simulink model "HVAC_Model"  (R2017b)
settings: Solver=VariableStepAuto  StartTime=0.0  StopTime=260  RelTol=1e-3
model workspace (MAT data in the model file):
  H_Speed = 3600
  H_limit = 2500
  L_limit = 0
  inputVoltage = 5
  nBitConverter = 10
undefined symbols (not defined in the file): sigbuilder_block
libraries: simulink x1
settings Model: Creator=ECoDe_user11  LastModifiedBy=ECoDe_user11
settings DebuggingCC: SignalInfNanChecking=warning  ParameterUnderflowMsg=warning  UniqueDataStoreMsg=warning
settings ConfigComp: CovEnable=on  RecordCoverage=on  CovMetricSettings=dcmwe  CovModelRefEnable=on

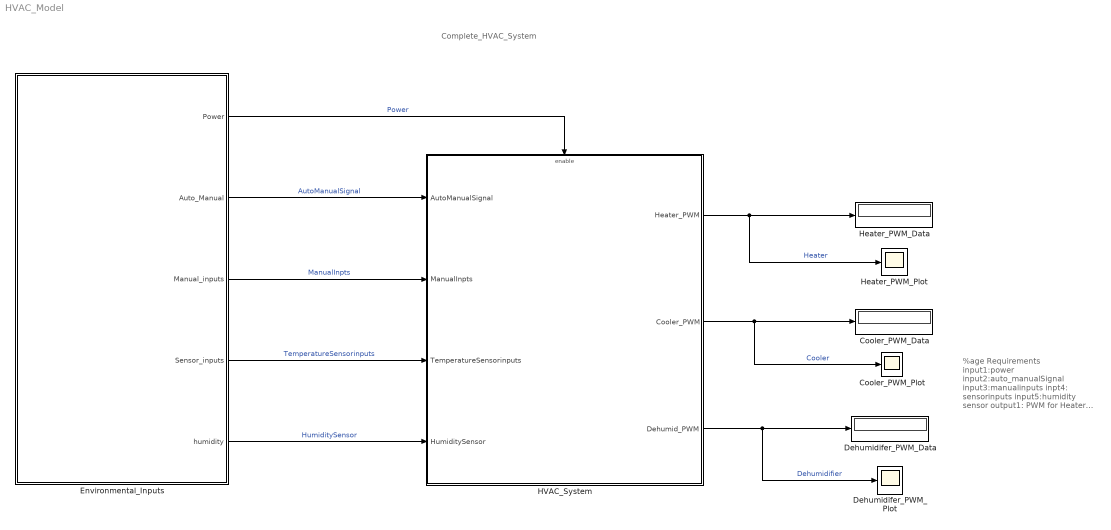
== system HVAC_Model ==
  note: Complete_HVAC_System
  note: %age Requirements
      |
      | input1:power
      | input2:auto_manualSignal
      | input3:manualinputs
      | inpt4: sensorinputs
      | input5:humidity sensor
      | output1: PWM for Heater
      | output1: PWM for Cooler
      | output1: PWM for Dehumidifier
  Cooler_PWM_Data : Display
  Cooler_PWM_Plot : Scope
  Dehumidifer_PWM_Data : Display
  Dehumidifer_PWM_Plot : Scope
  Environmental_Inputs : Subsystem  Tag=STV Subsys  LoadFcn=sigbuilder_block('load',[437.25 159 550.5 363.75 ]);  StartFcn=sigbuilder_block('start');  StopFcn=sigbuilder_block('stop');  ClipboardFcn=sigbuilder_block('clipboard');  mask(Sigbuilder block){tuvar=[0:10]}
      mask help: Simulink:masks:SigbuilderBlock_MD
      mask init:
      | if ~strcmp(get_param(bdroot(gcbh),'SimulationStatus'),'stopped') tuvar = sigbuilder_block('maskInit'); end
      settings: CopyFcn=sigbuilder_block('copy');  DeleteFcn=sigbuilder_block('delete');  ModelCloseFcn=sigbuilder_block('modelClose');  PreSaveFcn=sigbuilder_block('preSave');  PauseFcn=sigbuilder_block('pause');  ContinueFcn=sigbuilder_block('continue');  NameChangeFcn=sigbuilder_block('namechange');  OpenFcn=sigbuilder_block('open',[437.25 159 550.5 363.75 ]);  CloseFcn=sigbuilder_block('close');
      mask Display: plot(0, 0, 100, 100,[2, 2, 32, 32, 2], [68, 8, 8, 68, 68],[32, 2], [38, 38], [32, 19, 2],[53, 60, 44], [32, 17, 17, 2],[16, 16, 31, 31]);txt = getActiveGroup(gcbh);text(2, 100, txt,'verticalAlignment', 'top');
  HVAC_System : Subsystem
  Heater_PWM_Data : Display
  Heater_PWM_Plot : Scope
  wires:
  Environmental_Inputs/2(Auto_Manual) -> HVAC_System/1(AutoManualSignal)  "AutoManualSignal"
  Environmental_Inputs/3(Manual_inputs) -> HVAC_System/2(ManualInpts)  "ManualInpts"
  Environmental_Inputs/4(Sensor_inputs) -> HVAC_System/3(TemperatureSensorinputs)  "TemperatureSensorinputs"
  Environmental_Inputs/1(Power) -> HVAC_System/Enable  "Power"
  HVAC_System/1(Heater_PWM) -> Heater_PWM_Plot/1, Heater_PWM_Data/1  "Heater"
  HVAC_System/3(Dehumid_PWM) -> Dehumidifer_PWM_Plot/1, Dehumidifer_PWM_Data/1  "Dehumidifier"
  Environmental_Inputs/5(humidity) -> HVAC_System/4(HumiditySensor)  "HumiditySensor"
  HVAC_System/2(Cooler_PWM) -> Cooler_PWM_Plot/1, Cooler_PWM_Data/1  "Cooler"

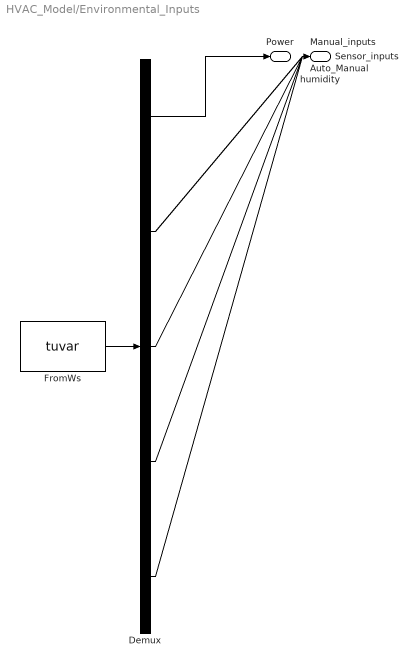
== system HVAC_Model/Environmental_Inputs ==
  Demux : Demux  Tag=STV Demux  Outputs=5
  FromWs : FromWorkspace  Tag=STV FromWs  VariableName=tuvar  SampleTime=0
      SigBuilderData=|
      | common.afterFinalStr = 'Extrapolate'
      | common.sampleTime = 0
      | dataSet.timeRange = [0 258]
      | dataSet.name = 'Sheet1'
      | sbobj.Name = 'Signal Builder'
      | sbobj.Groups.Name = 'Sheet1'
      | sbobj.Groups.Signals(1).Name = 'Power'
      | sbobj.Groups.Signals(1).XData = [0 1 2 3 4 5 6 7 8 9 10 11 12 13 14 15 16 17 18 19 20 21 22 23 24 25 26 27 28 29 30 31 32 33 34 35 36 37 38 39 40 41 42 43 44 45 46 47 48 49 50 51 52 53 54 55 56 57 58 59 60 61 62 63 64 65 66 67 68 69 70 71 72 73 74 75 76 77 78 79 80 81 82 83 84 85 86 87 88 89 90 91 92 93 94 95 96 97 98 99 100 101 102 103 104 105 106 107 108 109 110 111 112 113 114 115 116 117 118 119 120 121 122 123 124 125 126 127 128 129 130 131 132 133 134 135 136 137 138 139 140 141 142 143 144 145 146 147 148 149 150 151 152 153 154 155 156 157 158 159 160 161 162 163 164 165 166 167 168 169 170 171 172 173 174 175 176 177 178 179 180 181 182 183 184 185 186 187 188 189 190 191 192 193 194 195 196 197 198 199 200 201 202 203 204 205 206 207 208 209 210 211 212 213 214 215 216 217 218 219 220 221 222 223 224 225 226 227 228 229 230 231 232 233 234 235 236 237 238 239 240 241 242 243 244 245 246 247 248 249 250 251 252 253 254 255 256 257 258]
      | sbobj.Groups.Signals(1).YData = [1 1 1 1 1 1 1 1 1 1 1 1 1 1 1 1 1 1 1 1 1 1 1 1 1 1 1 1 1 1 1 1 1 1 1 1 1 1 1 1 1 1 1 1 1 1 1 1 1 1 1 1 1 1 1 1 1 1 1 1 1 1 1 1 1 1 1 1 1 1 1 1 0 0 0 0 0 0 0 1 1 1 1 1 1 1 1 1 1 1 1 1 1 1 1 1 1 1 1 1 1 1 1 1 1 1 1 1 1 1 1 1 1 1 1 1 1 1 1 1 1 1 1 1 1 1 1 1 1 1 1 1 1 1 1 1 1 1 1 1 1 1 1 1 1 1 1 1 1 1 1 1 1 1 1 1 1 1 1 1 1 1 1 1 1 1 1 1 1 1 1 1 1 1 1 1 1 1 1 1 1 1 1 1 1 1 1 1 1 1 1 1 1 1 1 1 1 1 1 1 1 1 1 1 1 1 1 1 1 1 1 1 1 1 1 1 1 1 1 1 1 1 1 1 1 1 1 1 1 1 1 1 1 1 1 1 1 1 1 1 1 1 1 1 1 1 1 1 1 1 1 1 1 1 1 1 1 1 1]
      | sbobj.Groups.Signals(2).Name = 'Auto_Manual'
      | sbobj.Groups.Signals(2).XData = [0 1 2 3 4 5 6 7 8 9 10 11 12 13 14 15 16 17 18 19 20 21 22 23 24 25 26 27 28 29 30 31 32 33 34 35 36 37 38 39 40 41 42 43 44 45 46 47 48 49 50 51 52 53 54 55 56 57 58 59 60 61 62 63 64 65 66 67 68 69 70 71 72 73 74 75 76 77 78 79 80 81 82 83 84 85 86 87 88 89 90 91 92 93 94 95 96 97 98 99 100 101 102 103 104 105 106 107 108 109 110 111 112 113 114 115 116 117 118 119 120 121 122 123 124 125 126 127 128 129 130 131 132 133 134 135 136 137 138 139 140 141 142 143 144 145 146 147 148 149 150 151 152 153 154 155 156 157 158 159 160 161 162 163 164 165 166 167 168 169 170 171 172 173 174 175 176 177 178 179 180 181 182 183 184 185 186 187 188 189 190 191 192 193 194 195 196 197 198 199 200 201 202 203 204 205 206 207 208 209 210 211 212 213 214 215 216 217 218 219 220 221 222 223 224 225 226 227 228 229 230 231 232 233 234 235 236 237 238 239 240 241 242 243 244 245 246 247 248 249 250 251 252 253 254 255 256 257 258]
      | sbobj.Groups.Signals(2).YData = [0 0 0 0 0 0 0 0 0 0 0 0 0 0 0 0 0 0 0 0 0 1 1 1 1 1 1 1 1 1 1 1 1 1 1 1 1 1 1 1 1 1 1 1 1 1 1 1 1 1 1 1 1 1 1 1 1 1 1 1 1 1 1 1 1 1 1 1 1 1 1 1 1 1 1 0 0 0 0 1 1 1 1 1 1 1 1 1 1 1 1 1 1 1 1 1 1 1 1 1 1 1 1 1 1 1 1 1 1 1 1 1 1 1 1 1 1 1 1 1 1 1 1 1 1 1 1 1 1 1 1 1 1 1 1 1 1 1 1 1 1 1 1 1 1 1 1 1 1 1 1 1 1 1 1 1 1 1 1 1 1 1 1 1 1 1 1 1 1 1 1 1 1 1 1 1 1 1 1 1 1 1 1 1 1 1 1 1 1 1 1 1 1 1 1 1 1 1 1 1 1 1 1 1 1 1 1 1 1 1 1 1 1 1 1 1 1 1 1 1 1 1 1 1 1 1 1 1 1 1 1 1 1 1 1 1 1 1 1 1 1 1 1 1 1 1 1 1 1 1 1 1 1 1 1 1 1 1 1]
      | sbobj.Groups.Signals(3).Name = 'Manual_inputs'
      | sbobj.Groups.Signals(3).XData = [0 1 2 3 4 5 6 7 8 9 10 11 12 13 14 15 16 17 18 19 20 21 22 23 24 25 26 27 28 29 30 31 32 33 34 35 36 37 38 39 40 41 42 43 44 45 46 47 48 49 50 51 52 53 54 55 56 57 58 59 60 61 62 63 64 65 66 67 68 69 70 71 72 73 74 75 76 77 78 79 80 81 82 83 84 85 86 87 88 89 90 91 92 93 94 95 96 97 98 99 100 101 102 103 104 105 106 107 108 109 110 111 112 113 114 115 116 117 118 119 120 121 122 123 124 125 126 127 128 129 130 131 132 133 134 135 136 137 138 139 140 141 142 143 144 145 146 147 148 149 150 151 152 153 154 155 156 157 158 159 160 161 162 163 164 165 166 167 168 169 170 171 172 173 174 175 176 177 178 179 180 181 182 183 184 185 186 187 188 189 190 191 192 193 194 195 196 197 198 199 200 201 202 203 204 205 206 207 208 209 210 211 212 213 214 215 216 217 218 219 220 221 222 223 224 225 226 227 228 229 230 231 232 233 234 235 236 237 238 239 240 241 242 243 244 245 246 247 248 249 250 251 252 253 254 255 256 257 258]
      | sbobj.Groups.Signals(3).YData = [14 15 16 17 18 19 20 21 22 23 24 25 26 27 28 29 30 31 32 33 34 0 1 2 3 4 5 6 7 8 9 10 11 12 13 14 15 16 17 18 19 20 21 22 23 24 25 26 27 28 29 30 31 32 33 34 35 36 37 38 39 40 41 42 43 44 45 46 47 48 49 50 17 18 19 20 21 22 23 24 25 26 27 27 27 27 27 27 27 27 27 27 27 27 27 27 27 27 27 27 27 27 27 27 27 27 27 27 27 27 27 27 27 27 27 27 27 27 27 27 27 27 27 27 27 27 27 27 27 27 27 27 27 27 24 25 26 27 20 20 20 20 20 20 20 20 20 20 20 20 20 20 20 20 20 20 20 20 20 20 20 20 20 20 20 20 20 20 20 20 20 20 20 20 20 20 20 20 20 20 20 20 20 20 20 20 20 20 20 20 20 20 20 20 20 20 20 20 20 20 20 20 20 20 20 20 20 20 20 20 20 20 20 20 20 20 20 20 20 20 20 20 20 20 20 20 20 20 20 20 20 20 20 20 20 20 20 20 20 20 20 20 20 20 20 20 20 20 20 20 20 20 20 20 20 20 20 20 20]
      | sbobj.Groups.Signals(4).Name = 'Sensor_inputs'
      | sbobj.Groups.Signals(4).XData = [0 1 2 3 4 5 6 7 8 9 10 11 12 13 14 15 16 17 18 19 20 21 22 23 24 25 26 27 28 29 30 31 32 33 34 35 36 37 38 39 40 41 42 43 44 45 46 47 48 49 50 51 52 53 54 55 56 57 58 59 60 61 62 63 64 65 66 67 68 69 70 71 72 73 74 75 76 77 78 79 80 81 82 83 84 85 86 87 88 89 90 91 92 93 94 95 96 97 98 99 100 101 102 103 104 105 106 107 108 109 110 111 112 113 114 115 116 117 118 119 120 121 122 123 124 125 126 127 128 129 130 131 132 133 134 135 136 137 138 139 140 141 142 143 144 145 146 147 148 149 150 151 152 153 154 155 156 157 158 159 160 161 162 163 164 165 166 167 168 169 170 171 172 173 174 175 176 177 178 179 180 181 182 183 184 185 186 187 188 189 190 191 192 193 194 195 196 197 198 199 200 201 202 203 204 205 206 207 208 209 210 211 212 213 214 215 216 217 218 219 220 221 222 223 224 225 226 227 228 229 230 231 232 233 234 235 236 237 238 239 240 241 242 243 244 245 246 247 248 249 250 251 252 253 254 255 256 257 258]
      | sbobj.Groups.Signals(4).YData = [0.1 0.2 0.3 0.4 0.5 0.6 0.7 0.8 0.9 1 1.1 1.2 1.3 1.4 1.5 1.6 1.7 1.8 1.9 2 2.1 0.9 0.89 0.88 0.87 0.86 0.85 0.84 0.83 0.82 0.81 0.8 0.79 0.78 0.77 0.76 0.75 0.74 0.73 0.72 0.71 0.7 0.69 0.68 0.67 0.66 0.65 0.64 0.63 0.62 0.61 0.6 0.59 0.58 0.57 0.56 0.55 0.54 0.53 0.52 0.51 0.5 0.49 0.48 0.47 0.46 0.45 0.44 0.43 0.42 0.41 0.4 0.1 0.2 0.3 0.4 0.5 0.6 0.7 0.71 0.71 0.71 0.71 0.4 0.41 0.42 0.43 0.44 0.45 0.46 0.47 0.48 0.49 0.5 0.51 0.52 0.53 0.54 0.55 0.56 0.57 0.58 0.59 0.6 0.61 0.62 0.63 0.64 0.65 0.66 0.67 0.68 0.69 0.7 0.71 0.72 0.73 0.74 0.75 0.76 0.77 0.78 0.79 0.8 0.81 0.82 0.83 0.84 0.85 0.86 0.87 0.88 0.89 0.9 0.71 0.71 0.71 0.71 0.71 0.71 0.8 0.71 0.69 0.7 0.71 0.7 0.68 0.71 0.7 0.68 0.63 0.71 0.7 0.68 0.63 0.58 0.71 0.7 0.68 0.63 0.58 0.53 0.71 0.7 0.68 0.63 0.58 0.53 0.48 0.71 0.7 0.68 0.63 0.58 0.53 0.48 0.43 0.71 0.7 0.68 0.63 0.58 0.53 0.48 0.43 0.38 0.71 0.73 0.71 0.73 0.75 0.71 0.73 0.75 0.76 0.71 0.73 0.75 0.76 0.79 0.71 0.73 0.75 0.76 0.79 0.81 0.71 0.73 0.75 0.76 0.79 0.81 0.83 0.71 0.73 0.75 0.76 0.79 0.81 0.83 0.84 0.71 0.73 0.75 0.76 0.79 0.81 0.83 0.84 0.86 0.71 0.73 0.75 0.76 0.79 0.81 0.83 0.84 0.86 0.88 0.71 0.73 0.75 0.76 0.79 0.81 0.83 0.84 0.86 0.88 0.86 0.84 0.83 0.81 0.79 0.76 0.75 0.73 0.71]
      | sbobj.Groups.Signals(5).Name = 'humidity'
      | sbobj.Groups.Signals(5).XData = [0 1 2 3 4 5 6 7 8 9 10 11 12 13 14 15 16 17 18 19 20 21 22 23 24 25 26 27 28 29 30 31 32 33 34 35 36 37 38 39 40 41 42 43 44 45 46 47 48 49 50 51 52 53 54 55 56 57 58 59 60 61 62 63 64 65 66 67 68 69 70 71 72 73 74 75 76 77 78 79 80 81 82 83 84 85 86 87 88 89 90 91 92 93 94 95 96 97 98 99 100 101 102 103 104 105 106 107 108 109 110 111 112 113 114 115 116 117 118 119 120 121 122 123 124 125 126 127 128 129 130 131 132 133 134 135 136 137 138 139 140 141 142 143 144 145 146 147 148 149 150 151 152 153 154 155 156 157 158 159 160 161 162 163 164 165 166 167 168 169 170 171 172 173 174 175 176 177 178 179 180 181 182 183 184 185 186 187 188 189 190 191 192 193 194 195 196 197 198 199 200 201 202 203 204 205 206 207 208 209 210 211 212 213 214 215 216 217 218 219 220 221 222 223 224 225 226 227 228 229 230 231 232 233 234 235 236 237 238 239 240 241 242 243 244 245 246 247 248 249 250 251 252 253 254 255 256 257 258]
      | sbobj.Groups.Signals(5).YData = [0 1 2 3 4 5 6 7 8 9 10 11 12 13 14 15 16 17 18 19 20 21 22 23 24 25 26 27 28 29 30 31 32 33 34 35 36 37 38 39 40 41 42 43 44 45 46 47 48 49 50 51 52 53 54 55 56 57 58 59 60 61 62 63 64 65 66 67 68 69 70 71 72 73 74 75 76 77 78 79 80 74 67 67 67 67 67 67 67 67 67 67 67 67 67 67 67 67 67 67 67 67 67 67 67 67 67 67 67 67 67 67 67 67 67 67 67 67 67 67 67 67 67 67 67 67 67 67 67 67 67 67 67 67 79 80 74 69 65 72 78 72 74 50 50 50 50 50 50 50 50 50 50 50 50 50 50 50 50 50 50 50 50 50 50 50 50 50 50 50 50 50 50 50 50 50 50 50 50 50 50 50 50 50 50 50 50 50 50 50 50 50 50 50 50 50 50 50 50 50 50 50 50 50 50 50 50 50 50 50 50 50 50 50 50 50 50 50 50 50 50 50 50 50 50 50 50 50 50 50 50 50 50 50 50 50 50 50 50 50 50 50 50 50 50 50 50 50 50 50 50 50 50 50 50 50 50 50 50]
      | sbobj.Groups.TimeRange = [0 133]
  Power : Outport  Tag=STV Outport
  Auto_Manual : Outport  Tag=STV Outport  Port=2
  Manual_inputs : Outport  Tag=STV Outport  Port=3
  Sensor_inputs : Outport  Tag=STV Outport  Port=4
  humidity : Outport  Tag=STV Outport  Port=5
  wires:
  Demux/1 -> Power/1
  FromWs/1 -> Demux/1
  Demux/2 -> Auto_Manual/1
  Demux/3 -> Manual_inputs/1
  Demux/4 -> Sensor_inputs/1
  Demux/5 -> humidity/1

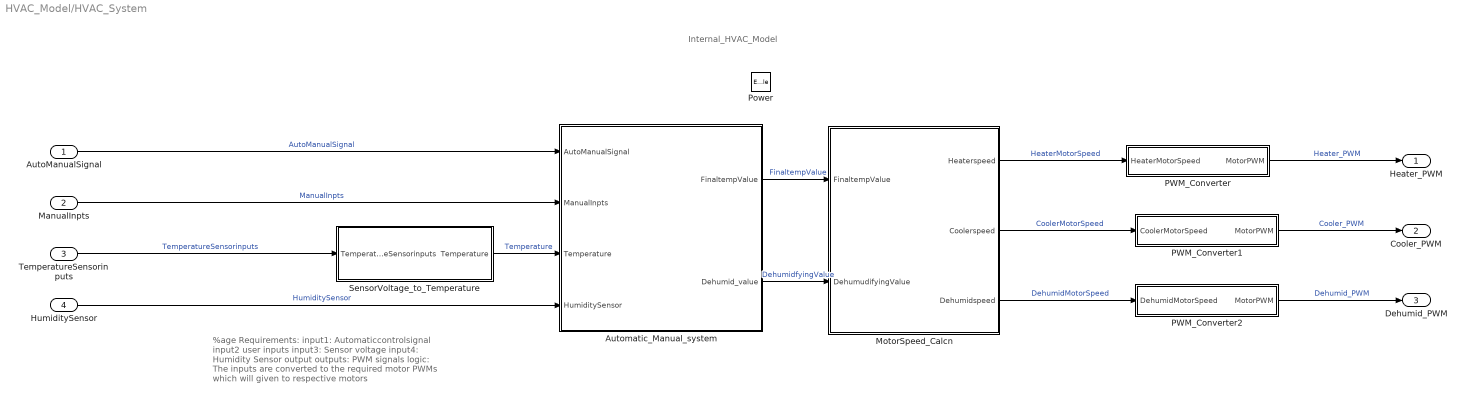
== system HVAC_Model/HVAC_System ==
  note: Internal_HVAC_Model
  note: %age Requirements:
      |
      | input1: Automaticcontrolsignal
      | input2 user inputs
      | input3: Sensor voltage
      | input4: Humidity Sensor output
      | outputs: PWM signals
      | logic: The inputs are converted to the required
      | motor PWMs which will given to respective motors
  AutoManualSignal : Inport
  ManualInpts : Inport  Port=2
  TemperatureSensorinputs : Inport  Port=3
  HumiditySensor : Inport  Port=4
  Power : EnablePort
  Automatic_Manual_system : Subsystem
  MotorSpeed_Calcn : Subsystem
  PWM_Converter : Subsystem
  PWM_Converter1 : Subsystem
  PWM_Converter2 : Subsystem
  SensorVoltage_to_Temperature : Subsystem
  Heater_PWM : Outport
  Cooler_PWM : Outport  Port=2
  Dehumid_PWM : Outport  Port=3
  wires:
  Automatic_Manual_system/2(Dehumid_value) -> MotorSpeed_Calcn/2(DehumudifyingValue)  "DehumidfyingValue"
  Automatic_Manual_system/1(FinaltempValue) -> MotorSpeed_Calcn/1(FinaltempValue)  "FinaltempValue"
  PWM_Converter1/1(MotorPWM) -> Cooler_PWM/1  "Cooler_PWM"
  TemperatureSensorinputs/1 -> SensorVoltage_to_Temperature/1(TemperatureSensorinputs)  "TemperatureSensorinputs"
  ManualInpts/1 -> Automatic_Manual_system/2(ManualInpts)  "ManualInpts"
  PWM_Converter/1(MotorPWM) -> Heater_PWM/1  "Heater_PWM"
  SensorVoltage_to_Temperature/1(Temperature) -> Automatic_Manual_system/3(Temperature)  "Temperature"
  PWM_Converter2/1(MotorPWM) -> Dehumid_PWM/1  "Dehumid_PWM"
  MotorSpeed_Calcn/2(Coolerspeed) -> PWM_Converter1/1(CoolerMotorSpeed)  "CoolerMotorSpeed"
  MotorSpeed_Calcn/1(Heaterspeed) -> PWM_Converter/1(HeaterMotorSpeed)  "HeaterMotorSpeed"
  AutoManualSignal/1 -> Automatic_Manual_system/1(AutoManualSignal)  "AutoManualSignal"
  MotorSpeed_Calcn/3(Dehumidspeed) -> PWM_Converter2/1(DehumidMotorSpeed)  "DehumidMotorSpeed"
  HumiditySensor/1 -> Automatic_Manual_system/4(HumiditySensor)  "HumiditySensor"

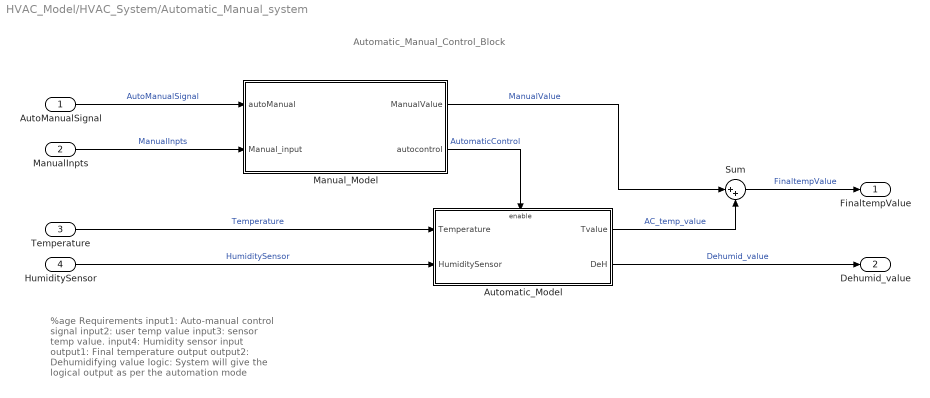
== system HVAC_Model/HVAC_System/Automatic_Manual_system ==
  note: Automatic_Manual_Control_Block
  note: %age Requirements
      |
      | input1: Auto-manual control signal
      | input2: user temp value
      | input3: sensor temp value.
      | input4: Humidity sensor input
      | output1: Final temperature output
      | output2: Dehumidifying value
      | logic: System will give the logical output as per
      | the automation mode
  AutoManualSignal : Inport
  ManualInpts : Inport  Port=2
  Temperature : Inport  Port=3
  HumiditySensor : Inport  Port=4
  Automatic_Model : Subsystem
  Manual_Model : Subsystem
  Sum : Sum  Inputs=|++
  FinaltempValue : Outport
  Dehumid_value : Outport  Port=2
  wires:
  Manual_Model/1(ManualValue) -> Sum/1  "ManualValue"
  Manual_Model/2(autocontrol) -> Automatic_Model/Enable  "AutomaticControl"
  AutoManualSignal/1 -> Manual_Model/1(autoManual)  "AutoManualSignal"
  ManualInpts/1 -> Manual_Model/2(Manual_input)  "ManualInpts"
  Sum/1 -> FinaltempValue/1  "FinaltempValue"
  Automatic_Model/1(Tvalue) -> Sum/2  "AC_temp_value"
  Temperature/1 -> Automatic_Model/1(Temperature)  "Temperature"
  Automatic_Model/2(DeH) -> Dehumid_value/1  "Dehumid_value"
  HumiditySensor/1 -> Automatic_Model/2(HumiditySensor)  "HumiditySensor"

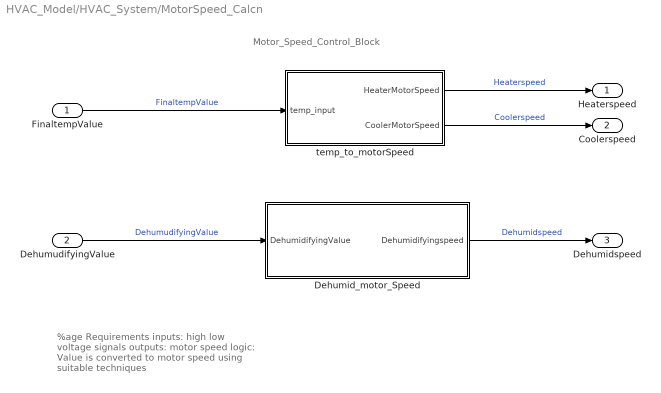
== system HVAC_Model/HVAC_System/MotorSpeed_Calcn ==
  note: Motor_Speed_Control_Block
  note: %age Requirements
      | inputs: high low voltage signals
      | outputs: motor speed
      | logic: Value is converted to motor speed
      | using suitable techniques
  FinaltempValue : Inport
  DehumudifyingValue : Inport  Port=2
  Dehumid_motor_Speed : Subsystem
  temp_to_motorSpeed : Subsystem
  Heaterspeed : Outport
  Coolerspeed : Outport  Port=2
  Dehumidspeed : Outport  Port=3
  wires:
  Dehumid_motor_Speed/1(Dehumidifyingspeed) -> Dehumidspeed/1  "Dehumidspeed"
  DehumudifyingValue/1 -> Dehumid_motor_Speed/1(DehumidifyingValue)  "DehumudifyingValue"
  temp_to_motorSpeed/1(HeaterMotorSpeed) -> Heaterspeed/1  "Heaterspeed"
  temp_to_motorSpeed/2(CoolerMotorSpeed) -> Coolerspeed/1  "Coolerspeed"
  FinaltempValue/1 -> temp_to_motorSpeed/1(temp_input)  "FinaltempValue"

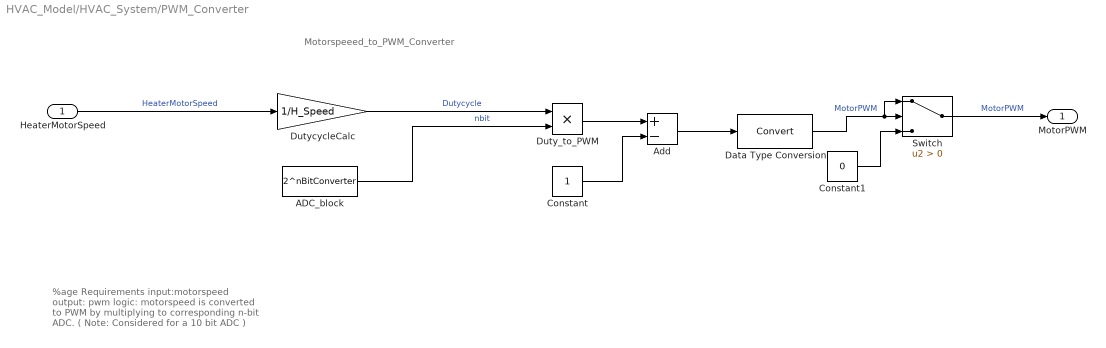
== system HVAC_Model/HVAC_System/PWM_Converter ==
  note: Motorspeeed_to_PWM_Converter
  note: %age Requirements
      |
      | input:motorspeed
      | output: pwm
      | logic: motorspeed is converted to PWM
      | by multiplying to corresponding n-bit ADC.
      | ( Note: Considered for a 10 bit ADC )
  HeaterMotorSpeed : Inport
  ADC_block : Constant  Value=2^nBitConverter
  Add : Sum  Inputs=+-
  Constant : Constant
  Constant1 : Constant  Value=0
  Data Type Conversion : DataTypeConversion
  Duty_to_PWM : Product
  DutycycleCalc : Gain  Gain=1/H_Speed
  Switch : Switch  Criteria=u2 > Threshold
  MotorPWM : Outport
  wires:
  HeaterMotorSpeed/1 -> DutycycleCalc/1  "HeaterMotorSpeed"
  ADC_block/1 -> Duty_to_PWM/2  "nbit"
  DutycycleCalc/1 -> Duty_to_PWM/1  "Dutycycle"
  Duty_to_PWM/1 -> Add/1
  Constant/1 -> Add/2
  Add/1 -> Data Type Conversion/1
  Data Type Conversion/1 -> Switch/1, Switch/2  "MotorPWM"
  Constant1/1 -> Switch/3
  Switch/1 -> MotorPWM/1  "MotorPWM"

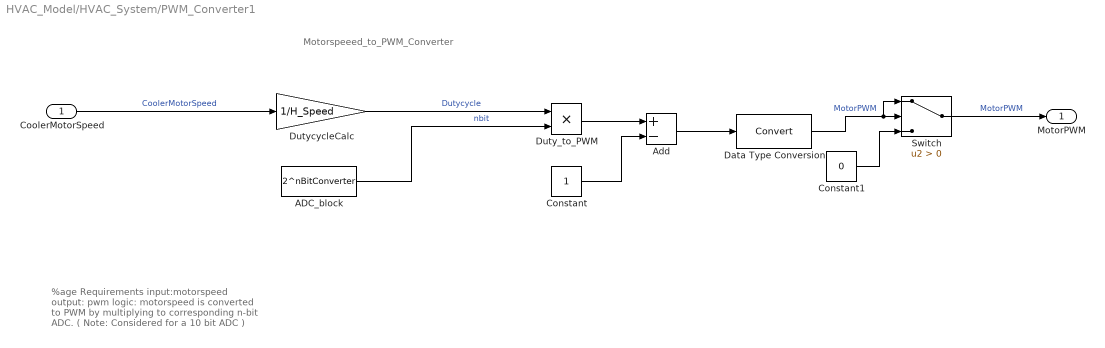
== system HVAC_Model/HVAC_System/PWM_Converter1 ==
  note: Motorspeeed_to_PWM_Converter
  note: %age Requirements
      |
      | input:motorspeed
      | output: pwm
      | logic: motorspeed is converted to PWM
      | by multiplying to corresponding n-bit ADC.
      | ( Note: Considered for a 10 bit ADC )
  CoolerMotorSpeed : Inport
  ADC_block : Constant  Value=2^nBitConverter
  Add : Sum  Inputs=+-
  Constant : Constant
  Constant1 : Constant  Value=0
  Data Type Conversion : DataTypeConversion
  Duty_to_PWM : Product
  DutycycleCalc : Gain  Gain=1/H_Speed
  Switch : Switch  Criteria=u2 > Threshold
  MotorPWM : Outport
  wires:
  CoolerMotorSpeed/1 -> DutycycleCalc/1  "CoolerMotorSpeed"
  ADC_block/1 -> Duty_to_PWM/2  "nbit"
  DutycycleCalc/1 -> Duty_to_PWM/1  "Dutycycle"
  Duty_to_PWM/1 -> Add/1
  Constant/1 -> Add/2
  Add/1 -> Data Type Conversion/1
  Data Type Conversion/1 -> Switch/1, Switch/2  "MotorPWM"
  Constant1/1 -> Switch/3
  Switch/1 -> MotorPWM/1  "MotorPWM"

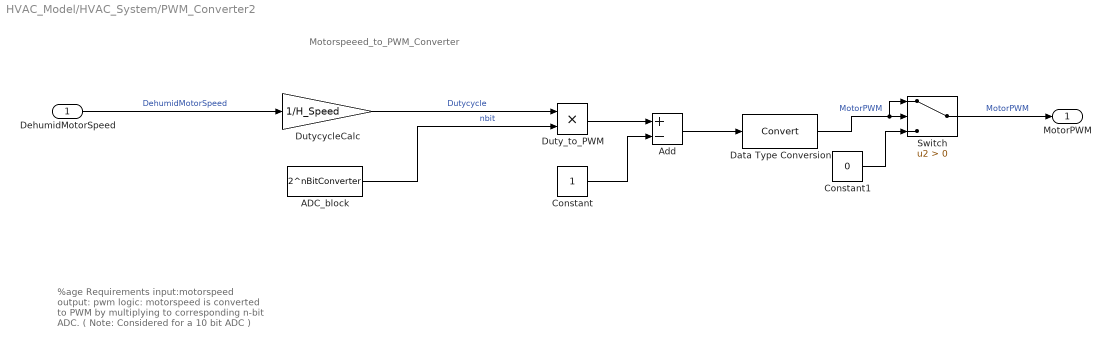
== system HVAC_Model/HVAC_System/PWM_Converter2 ==
  note: Motorspeeed_to_PWM_Converter
  note: %age Requirements
      |
      | input:motorspeed
      | output: pwm
      | logic: motorspeed is converted to PWM
      | by multiplying to corresponding n-bit ADC.
      | ( Note: Considered for a 10 bit ADC )
  DehumidMotorSpeed : Inport
  ADC_block : Constant  Value=2^nBitConverter
  Add : Sum  Inputs=+-
  Constant : Constant
  Constant1 : Constant  Value=0
  Data Type Conversion : DataTypeConversion
  Duty_to_PWM : Product
  DutycycleCalc : Gain  Gain=1/H_Speed
  Switch : Switch  Criteria=u2 > Threshold
  MotorPWM : Outport
  wires:
  DehumidMotorSpeed/1 -> DutycycleCalc/1  "DehumidMotorSpeed"
  ADC_block/1 -> Duty_to_PWM/2  "nbit"
  DutycycleCalc/1 -> Duty_to_PWM/1  "Dutycycle"
  Duty_to_PWM/1 -> Add/1
  Constant/1 -> Add/2
  Add/1 -> Data Type Conversion/1
  Data Type Conversion/1 -> Switch/1, Switch/2  "MotorPWM"
  Constant1/1 -> Switch/3
  Switch/1 -> MotorPWM/1  "MotorPWM"

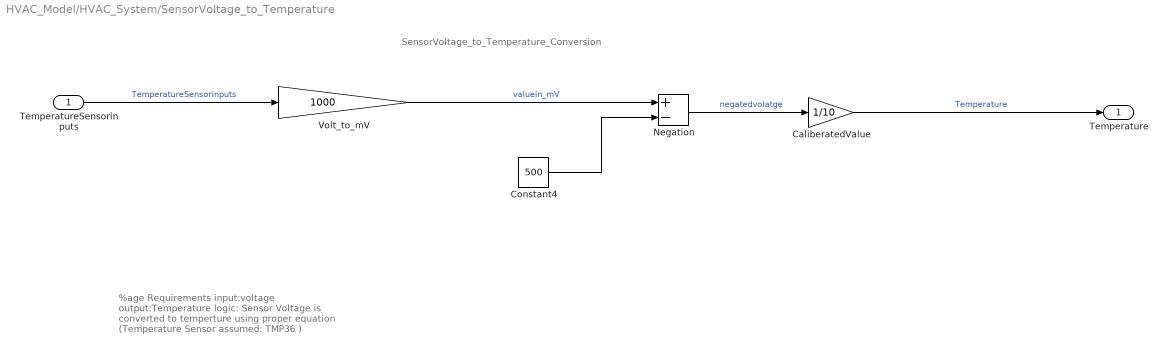
== system HVAC_Model/HVAC_System/SensorVoltage_to_Temperature ==
  note: %age Requirements
      |
      | input:voltage
      | output:Temperature
      | logic: Sensor Voltage is converted to temperture
      | using proper equation
      | (Temperature Sensor assumed: TMP36 )
  note: SensorVoltage_to_Temperature_Conversion
  TemperatureSensorinputs : Inport
  CaliberatedValue : Gain  Gain=1/10
  Constant4 : Constant  Value=500
  Negation : Sum  Inputs=+-
  Volt_to_mV : Gain  Gain=1000
  Temperature : Outport
  wires:
  Volt_to_mV/1 -> Negation/1  "valuein_mV"
  Constant4/1 -> Negation/2
  CaliberatedValue/1 -> Temperature/1  "Temperature"
  TemperatureSensorinputs/1 -> Volt_to_mV/1  "TemperatureSensorinputs"
  Negation/1 -> CaliberatedValue/1  "negatedvolatge"

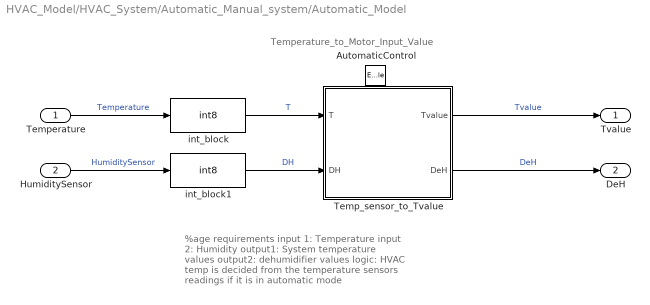
== system HVAC_Model/HVAC_System/Automatic_Manual_system/Automatic_Model ==
  note: Temperature_to_Motor_Input_Value
  note: %age requirements
      |
      | input 1: Temperature
      | input 2: Humidity
      | output1: System temperature values
      | output2: dehumidifier values
      | logic:
      | HVAC temp is decided from the temperature
      | sensors readings if it is in automatic mode
  Temperature : Inport
  HumiditySensor : Inport  Port=2
  AutomaticControl : EnablePort
  Temp_sensor_to_Tvalue : Stateflow chart  TreatAsAtomicUnit=on
  int_block : DataTypeConversion  OutDataTypeStr=int8
  int_block1 : DataTypeConversion  OutDataTypeStr=int8
  Tvalue : Outport
  DeH : Outport  Port=2
  wires:
  Temp_sensor_to_Tvalue/1(Tvalue) -> Tvalue/1  "Tvalue"
  Temp_sensor_to_Tvalue/2(DeH) -> DeH/1  "DeH"
  Temperature/1 -> int_block/1  "Temperature"
  HumiditySensor/1 -> int_block1/1  "HumiditySensor"
  int_block/1 -> Temp_sensor_to_Tvalue/1(T)  "T"
  int_block1/1 -> Temp_sensor_to_Tvalue/2(DH)  "DH"

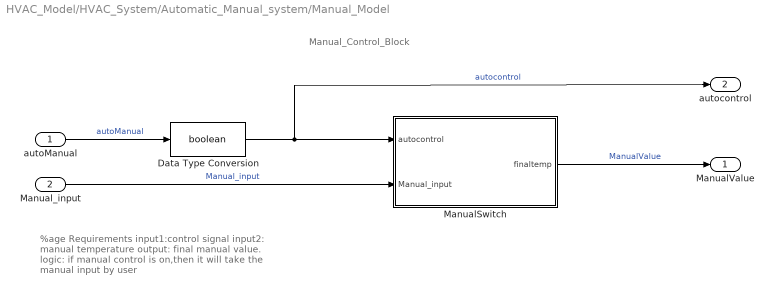
== system HVAC_Model/HVAC_System/Automatic_Manual_system/Manual_Model ==
  note: Manual_Control_Block
  note: %age Requirements
      |
      | input1:control signal
      | input2: manual temperature
      | output: final manual value.
      | logic: if manual control is on,then it will take the
      | manual input by user
  autoManual : Inport
  Manual_input : Inport  Port=2
  Data Type Conversion : DataTypeConversion  OutDataTypeStr=boolean
  ManualSwitch : Subsystem
  ManualValue : Outport
  autocontrol : Outport  Port=2
  wires:
  Data Type Conversion/1 -> autocontrol/1, ManualSwitch/1(autocontrol)  "autocontrol"
  autoManual/1 -> Data Type Conversion/1  "autoManual"
  Manual_input/1 -> ManualSwitch/2(Manual_input)  "Manual_input"
  ManualSwitch/1(finaltemp) -> ManualValue/1  "ManualValue"

== system HVAC_Model/HVAC_System/MotorSpeed_Calcn/Dehumid_motor_Speed ==
  note: Dehumidifier_Speed
  note: %age Requirements
      |
      | input: Dehumidfyingvalue
      | output: Motor speed
      | logic: Motor speed is given as
      | per the dehumidfying value
  DehumidifyingValue : Inport
  HighestMotorValue : Constant  Value=H_limit
  LowestMotorValue : Constant  Value=L_limit
  Switch : Switch  Criteria=u2 ~= 0
  Dehumidifyingspeed : Outport
  wires:
  HighestMotorValue/1 -> Switch/1  "HighestMotorspeed"
  LowestMotorValue/1 -> Switch/3  "lowerMotorSpeed"
  DehumidifyingValue/1 -> Switch/2  "DehumidifyingValue"
  Switch/1 -> Dehumidifyingspeed/1  "Dehumidifyingspeed"

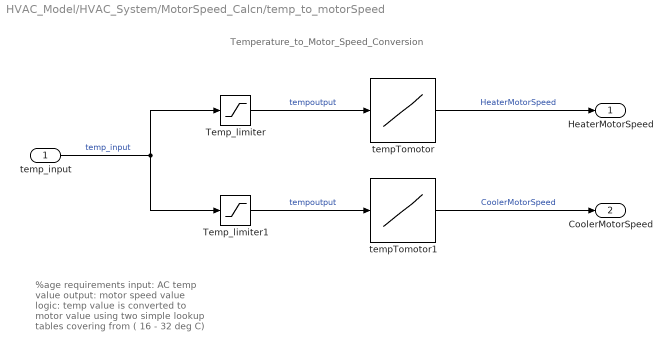
== system HVAC_Model/HVAC_System/MotorSpeed_Calcn/temp_to_motorSpeed ==
  note: %age requirements
      |
      | input: AC temp value
      | output: motor speed value
      | logic: temp value is converted to motor value using two simple lookup tables covering from ( 16 - 32 deg C)
  note: Temperature_to_Motor_Speed_Conversion
  temp_input : Inport
  Temp_limiter : Saturate  UpperLimit=32  LowerLimit=25
  Temp_limiter1 : Saturate  UpperLimit=26  LowerLimit=16
  tempTomotor : Lookup_n-D  NumberOfTableDimensions=1  BreakpointsForDimension1=[25:32]  Table=[0 500 1000 1500 2000 2500 3000 3600]  InternalRulePriority=Speed  RndMeth=Simplest  InputSameDT=on
  tempTomotor1 : Lookup_n-D  NumberOfTableDimensions=1  BreakpointsForDimension1=[16:26]  Table=[3600 3400 3200 2800 2400 2000 1600 1300 900 500 0]  InternalRulePriority=Speed  RndMeth=Simplest  InputSameDT=on
  HeaterMotorSpeed : Outport
  CoolerMotorSpeed : Outport  Port=2
  wires:
  Temp_limiter1/1 -> tempTomotor1/1  "tempoutput"
  Temp_limiter/1 -> tempTomotor/1  "tempoutput"
  temp_input/1 -> Temp_limiter1/1, Temp_limiter/1  "temp_input"
  tempTomotor/1 -> HeaterMotorSpeed/1  "HeaterMotorSpeed"
  tempTomotor1/1 -> CoolerMotorSpeed/1  "CoolerMotorSpeed"

== system HVAC_Model/HVAC_System/Automatic_Manual_system/Manual_Model/ManualSwitch ==
  note: %age Requirements
      |
      | input: voltage
      | input2: temperature
      | output: Final temp value
      | logic: Manual control for HVAC system
  note: Manual_Control_Subsystem
  autocontrol : Inport
  Manual_input : Inport  Port=2
  Bitwise Operator : simulink/Logic and Bit Operations/Bitwise Operator  logicop=NOT  UseBitMask=off  BitMask=bin2dec('11011001')  BitMaskRealWorld=Stored Integer
  Product : Product
  Saturation : Saturate  UpperLimit=32  LowerLimit=16
      settings: AttributesFormatString=%<LowerLimit>
  finaltemp : Outport
  wires:
  Bitwise Operator/1 -> Product/1  "manualControl"
  Manual_input/1 -> Saturation/1  "Manual_input"
  Saturation/1 -> Product/2  "limitedop"
  autocontrol/1 -> Bitwise Operator/1  "autocontrol"
  Product/1 -> finaltemp/1  "finaltemp"

== stateflow chart HVAC_Model/HVAC_System/Automatic_Manual_system/Automatic_Model/Temp_sensor_to_Tvalue ==
  note: TempValue_Select_Model
  state HeaterState
    en:
    DeH=0;
    Tvalue=26;
    state at_20
      en:
      Tvalue=26;
    state bet_15_20
      en:
      Tvalue=27;
    state bet_10_15
      en:
      Tvalue=28;
    state bet_0_5
      en:
      Tvalue=30;
    state bet_5_10
      en:
      Tvalue=29;
    state bet_n5_0
      en:
      Tvalue=31;
    state less_n5
      en:
      Tvalue=32;
    (default) -> at_20
    bet_15_20 -> at_20 [order 2] : [T>19]
    at_20 -> bet_15_20 : [T<20]
    bet_10_15 -> bet_15_20 [order 1] : [T>14]
    bet_15_20 -> bet_10_15 [order 1] : [T<15]
    bet_10_15 -> bet_5_10 [order 2] : [T<10]
    bet_5_10 -> bet_10_15 [order 2] : [T>9]
    bet_0_5 -> bet_5_10 [order 1] : [T>4]
    bet_5_10 -> bet_0_5 [order 1] : [T<5]
    bet_0_5 -> bet_n5_0 [order 2] : [T<0]
    bet_n5_0 -> bet_0_5 [order 2] : [T>-1]
    bet_n5_0 -> less_n5 [order 1] : [T<-5]
    less_n5 -> bet_n5_0 : [T>-6]
  state CoolerState
    en:
    DeH=0;
    Tvalue=25;
    state bet_23_24
      en:
      Tvalue=25;
    state bet_24_25
      en:
      Tvalue=24;
    state bet_25_27
      en:
      Tvalue=23;
    state bet_28_30
      en:
      Tvalue=21;
    state bet_27_28
      en:
      Tvalue=22;
    state bet_30_32
      en:
      Tvalue=20;
    state bet_32_33
      en:
      Tvalue=19;
    state bet_35_37
      en:
      Tvalue=17;
    state bet_33_35
      en:
      Tvalue=18;
    state grt_37
      en:
      Tvalue=16;
    (default) -> bet_23_24
    bet_24_25 -> bet_23_24 [order 2] : [T<25]
    bet_23_24 -> bet_24_25 : [T>24]
    bet_25_27 -> bet_24_25 [order 1] : [T<26]
    bet_24_25 -> bet_25_27 [order 1] : [T>25]
    bet_25_27 -> bet_27_28 [order 2] : [T>27]
    bet_27_28 -> bet_25_27 [order 2] : [T<28]
    bet_28_30 -> bet_27_28 [order 1] : [T<29]
    bet_27_28 -> bet_28_30 [order 1] : [T>28]
    bet_28_30 -> bet_30_32 [order 2] : [T>30]
    bet_30_32 -> bet_28_30 [order 2] : [T<31]
    bet_30_32 -> bet_32_33 [order 1] : [T>32]
    bet_32_33 -> bet_30_32 [order 1] : [T<33]
    bet_33_35 -> bet_32_33 [order 1] : [T<34]
    bet_32_33 -> bet_33_35 [order 2] : [T>33]
    bet_33_35 -> bet_35_37 [order 2] : [T>35]
    bet_35_37 -> bet_33_35 [order 2] : [T<36]
    grt_37 -> bet_35_37 : [T<38]
    bet_35_37 -> grt_37 [order 1] : [T>37]
  state Normal_temp
    state DehumifyingState
      en:
      DeH=1;
    state On_OffState
      en:
      DeH=0;
      Tvalue=0;
    (default) -> On_OffState
    On_OffState -> DehumifyingState : [DH>70]
    DehumifyingState -> On_OffState : [DH<70]
  note: %age Requirements:
      |
      | input:Temperuture
      | input 2: humidity
      | output1:Temperature Value
      | output2: Dehumidifier Value
  Normal_temp -> at_20 [order 2] : [T<21]
  Normal_temp -> bet_23_24 [order 1] : [T>22]
  HeaterState -> On_OffState : [T>20]
  (default) -> Normal_temp
  CoolerState -> On_OffState : [T<23]
  data: Tvalue output; DeH output; T input; DH input
